simulink subsystem "propagation"  (R2023b)
settings: Solver=VariableStepAuto  StartTime=0.0  StopTime=10.0  RelTol=1e-3
undefined symbols (not defined in the file or in its folder): P0, Propagation, R_sensor2body, x0
undefined symbols (not defined in the file): states_k
libraries: nav_lib x7
settings Model: Creator=brent  LastModifiedBy=brent

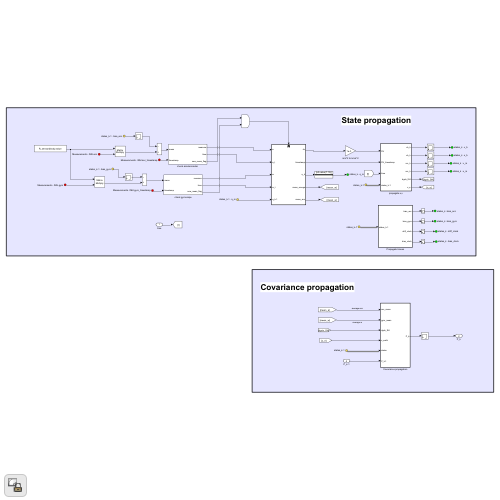
[thumbnail: Simulink's stored preview of the top-level diagram]
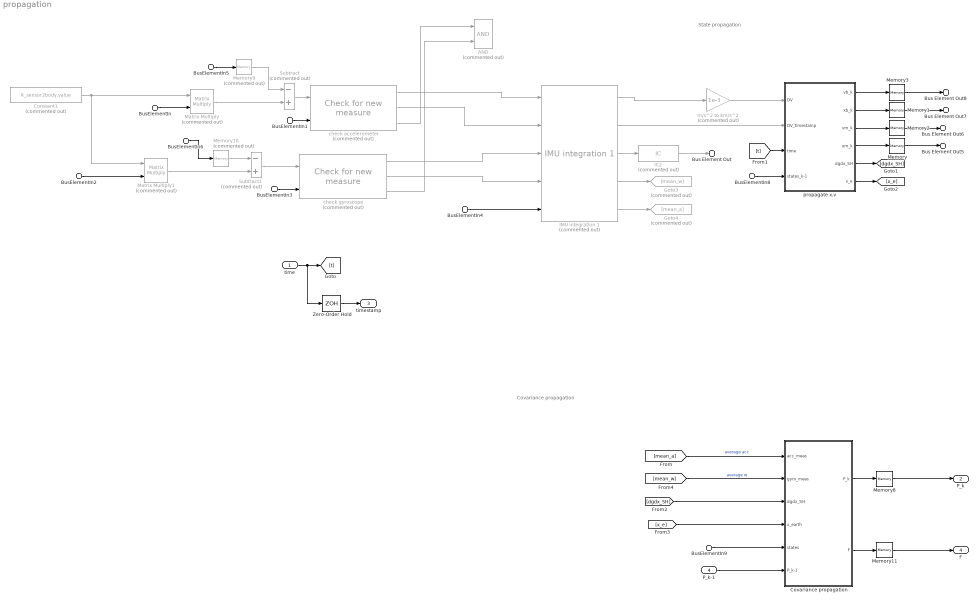
== system propagation ==
  note: State propagation
  note: Covariance propagation
  time : Inport
  BusElementIn1 : Inport  Port=2  PortName=Measurements  Element=IMU.acc_timestamp
  BusElementIn3 : Inport  Port=2  PortName=Measurements  Element=IMU.gyro_timestamp
  BusElementIn : Inport  Port=2  PortName=Measurements  Element=IMU.acc
  BusElementIn2 : Inport  Port=2  PortName=Measurements  Element=IMU.gyro
  BusElementIn8 : Inport  Port=3  PortName=states_k-1
  BusElementIn9 : Inport  Port=3  PortName=states_k-1
  BusElementIn4 : Inport  Port=3  PortName=states_k-1  Element=q_m
  BusElementIn5 : Inport  Port=3  PortName=states_k-1  Element=bias_acc
  BusElementIn6 : Inport  Port=3  PortName=states_k-1  Element=bias_gyro
  P_k-1 : Inport  Port=4
  AND : Logic  Commented=on  IconShape=distinctive  AllPortsSameDT=off  OutDataTypeStr=boolean
  Constant1 : Constant  Commented=on  Value=R_sensor2body.value
  Covariance propagation : Subsystem  TreatAsAtomicUnit=on  SystemSampleTime=1/Propagation.lf.value
  Goto3 : Goto  Commented=on  GotoTag=mean_w
  Goto4 : Goto  Commented=on  GotoTag=mean_a
  IC2 : InitialCondition  Commented=on  Value=x0.value(7:10)
  IMU integration 1 : nav_lib/IMU integration 1  Commented=on  q0=x0.value(7:10)  HF=Propagation.hf.value  LF=Propagation.lf.value
      settings: SourceProductName=Navigation library
  Matrix Multiply : Product  Commented=on  Multiplication=Matrix(*)
  Matrix Multiply1 : Product  Commented=on  Multiplication=Matrix(*)
  Memory : Memory  InitialCondition=x0.value(1:3)  InheritSampleTime=on
  Memory1 : Memory  InitialCondition=x0.value(11:13)  InheritSampleTime=on
  Memory10 : Memory  Commented=on  InitialCondition=x0.value(20:22)
  Memory11 : Memory  InitialCondition=eye(12)  InheritSampleTime=on
  Memory2 : Memory  InitialCondition=x0.value(4:6)  InheritSampleTime=on
  Memory3 : Memory  InitialCondition=x0.value(14:16)  InheritSampleTime=on
  Memory8 : Memory  InitialCondition=P0.value([1:6 10:15],[1:6 10:15])  InheritSampleTime=on
  Memory9 : Memory  Commented=on  InitialCondition=x0.value(17:19)
  Subtract : Sum  Commented=on  Inputs=-+
  Subtract1 : Sum  Commented=on  Inputs=-+
  Zero-Order Hold : ZeroOrderHold  SampleTime=1/Propagation.lf.value
  check accelerometer : nav_lib/Check for new measure  Commented=on  Ts=1/Propagation.hf.value
      settings: SourceProductName=Navigation library
  check gyroscope : nav_lib/Check for new measure  Commented=on  Ts=1/Propagation.hf.value
      settings: SourceProductName=Navigation library
  m/s^2 to km/s^2 : Gain  Commented=on  Gain=1e-3
  propagate x,v : Subsystem  TreatAsAtomicUnit=on  SystemSampleTime=1/Propagation.lf.value
  Bus Element Out5 : Outport  PortName=states_k  Element=x_m
  Bus Element Out6 : Outport  PortName=states_k  Element=v_m
  Bus Element Out : Outport  PortName=states_k  Element=q_m
  Bus Element Out7 : Outport  PortName=states_k  Element=x_b
  Bus Element Out8 : Outport  PortName=states_k  Element=v_b
  P_k : Outport  Port=2
  timestamp : Outport  Port=3
  F : Outport  Port=4
  wires:
  BusElementIn1/1 -> check accelerometer/2
  BusElementIn3/1 -> check gyroscope/2
  check accelerometer/3 -> AND/1
  check gyroscope/3 -> AND/2
  time/1 -> [t], Zero-Order Hold/1
  BusElementIn/1 -> Matrix Multiply/2
  Constant1/1 -> Matrix Multiply1/1, Matrix Multiply/1
  BusElementIn2/1 -> Matrix Multiply1/2
  Matrix Multiply/1 -> Subtract/2
  Subtract/1 -> check accelerometer/1
  BusElementIn5/1 -> Memory9/1
  m/s^2 to km/s^2/1 -> propagate x,v/1(DV)
  Subtract1/1 -> check gyroscope/1
  BusElementIn6/1 -> Memory10/1
  Matrix Multiply1/1 -> Subtract1/2
  [t] -> propagate x,v/3(time)
  BusElementIn8/1 -> propagate x,v/4(states_k-1)
  propagate x,v/4(xm_k) -> Memory/1
  propagate x,v/3(vm_k) -> Memory2/1
  propagate x,v/2(xb_k) -> Memory1/1
  propagate x,v/1(vb_k) -> Memory3/1
  Memory1/1 -> Bus Element Out7/1
  Memory/1 -> Bus Element Out5/1
  Memory2/1 -> Bus Element Out6/1
  Memory3/1 -> Bus Element Out8/1
  BusElementIn4/1 -> IMU integration 1/5
  IC2/1 -> Bus Element Out/1
  propagate x,v/5(dgdx_SH) -> [dgdx_SH]
  propagate x,v/6(x_e) -> [x_e]
  [dgdx_SH] -> Covariance propagation/3(dgdx_SH)
  [x_e] -> Covariance propagation/4(x_earth)
  BusElementIn9/1 -> Covariance propagation/5(states)
  P_k-1/1 -> Covariance propagation/6(P_k-1)
  IMU integration 1/4 -> Goto3/1
  [mean_w] -> Covariance propagation/2(gyro_meas)  "average w"
  [mean_a] -> Covariance propagation/1(acc_meas)  "average acc"
  check accelerometer/1 -> IMU integration 1/1
  check accelerometer/2 -> IMU integration 1/2
  check gyroscope/1 -> IMU integration 1/3
  check gyroscope/2 -> IMU integration 1/4
  IMU integration 1/1 -> m/s^2 to km/s^2/1
  IMU integration 1/3 -> IC2/1
  IMU integration 1/2 -> propagate x,v/2(DV_timestamp)
  IMU integration 1/5 -> Goto4/1
  Covariance propagation/1(P_k) -> Memory8/1
  Memory8/1 -> P_k/1
  Memory9/1 -> Subtract/1
  Memory10/1 -> Subtract1/1
  Zero-Order Hold/1 -> timestamp/1
  Covariance propagation/2(F) -> Memory11/1
  Memory11/1 -> F/1

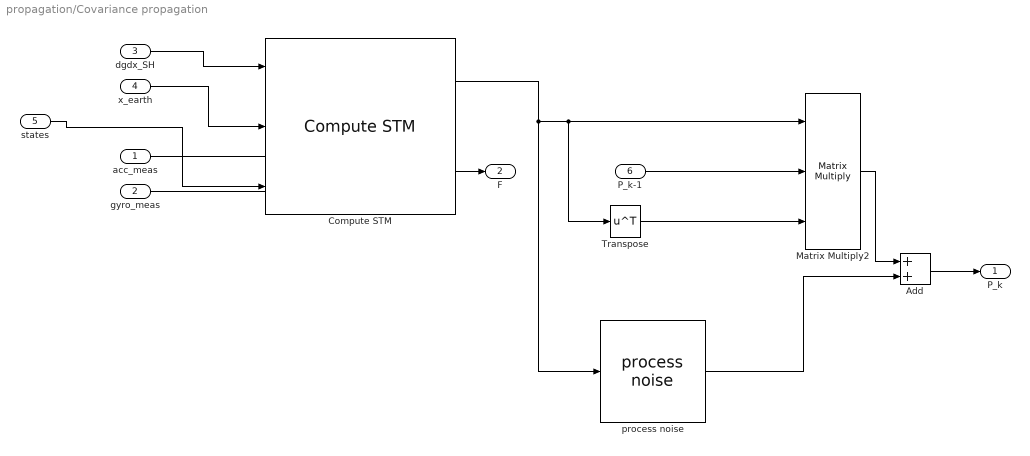
== system propagation/Covariance propagation ==
  acc_meas : Inport
  gyro_meas : Inport  Port=2
  dgdx_SH : Inport  Port=3
  x_earth : Inport  Port=4
  states : Inport  Port=5
  P_k-1 : Inport  Port=6
  Add : Sum
  Compute STM : nav_lib/Compute STM  dt=1/Propagation.lf.value  mu_e=Propagation.Earth.mu.value  mu_m=Propagation.Moon.mu.value  x0=x0.value
      settings: SourceProductName=Navigation library
  Matrix Multiply2 : Product  Inputs=3  Multiplication=Matrix(*)
  Transpose : Math  Operator=transpose
  process noise : nav_lib/process noise  Q=Q.value  R_sb=R_sensor2body.value  dt=1/Propagation.lf.value
      settings: SourceProductName=Navigation library
  P_k : Outport
  F : Outport  Port=2
  wires:
  process noise/1 -> Add/2
  Compute STM/2 -> F/1
  Add/1 -> P_k/1
  Matrix Multiply2/1 -> Add/1
  Compute STM/1 -> Transpose/1, Matrix Multiply2/1, process noise/1
  states/1 -> Compute STM/3
  x_earth/1 -> Compute STM/2
  dgdx_SH/1 -> Compute STM/1
  Transpose/1 -> Matrix Multiply2/3
  P_k-1/1 -> Matrix Multiply2/2
  gyro_meas/1 -> ?
  acc_meas/1 -> ?

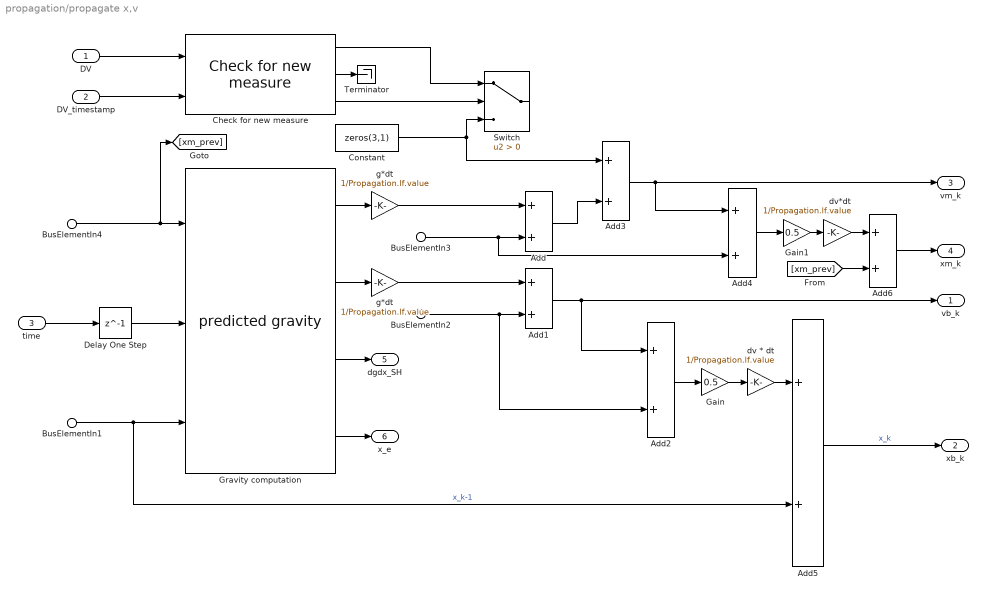
== system propagation/propagate x,v ==
  DV : Inport
  DV_timestamp : Inport  Port=2
  time : Inport  Port=3
  BusElementIn4 : Inport  Port=4  PortName=states_k-1  Element=x_m
  BusElementIn3 : Inport  Port=4  PortName=states_k-1  Element=v_m
  BusElementIn1 : Inport  Port=4  PortName=states_k-1  Element=x_b
  BusElementIn2 : Inport  Port=4  PortName=states_k-1  Element=v_b
  Add{,1..6} (7 alike) : Sum
  Check for new measure : nav_lib/Check for new measure  Ts=0
      settings: SourceProductName=Navigation library
  Constant : Constant  Value=zeros(3,1)  VectorParams1D=off
  Delay One Step : Delay  DelayLength=1
  Gain : Gain  Gain=0.5
  Gain1 : Gain  Gain=0.5
  Gravity computation : nav_lib/predicted gravity  date=StartDate  Earth=Propagation.Earth  Moon=Propagation.Moon
      settings: SourceProductName=Navigation library
  Switch : Switch  Criteria=u2 > Threshold  SaturateOnIntegerOverflow=off  InputSameDT=off
  Terminator : Terminator
  dv * dt : Gain  Gain=1/Propagation.lf.value
  dv*dt : Gain  Gain=1/Propagation.lf.value
  g*dt : Gain  Gain=1/Propagation.lf.value
  "g*dt " : Gain  Gain=1/Propagation.lf.value
  vb_k : Outport
  xb_k : Outport  Port=2
  vm_k : Outport  Port=3
  xm_k : Outport  Port=4
  dgdx_SH : Outport  Port=5
  x_e : Outport  Port=6
  wires:
  Delay One Step/1 -> Gravity computation/2
  dv*dt/1 -> Add6/1
  Gain1/1 -> dv*dt/1
  dv * dt/1 -> Add5/1
  Gravity computation/4 -> x_e/1
  Gravity computation/3 -> dgdx_SH/1
  Add6/1 -> xm_k/1
  [xm_prev] -> Add6/2
  Add5/1 -> xb_k/1  "x_k"
  Gain/1 -> dv * dt/1
  BusElementIn1/1 -> Add5/2, Gravity computation/3  "x_k-1"
  BusElementIn4/1 -> Gravity computation/1, [xm_prev]
  time/1 -> Delay One Step/1
  Add4/1 -> Gain1/1
  BusElementIn3/1 -> Add/2, Add4/2
  Add3/1 -> vm_k/1, Add4/1
  "g*dt "/1 -> Add/1
  Constant/1 -> Switch/3, Add3/1
  Check for new measure/1 -> Switch/1
  Add/1 -> Add3/2
  Add2/1 -> Gain/1
  BusElementIn2/1 -> Add1/2, Add2/2
  Add1/1 -> vb_k/1, Add2/1
  Check for new measure/3 -> Switch/2
  g*dt/1 -> Add1/1
  Gravity computation/2 -> g*dt/1
  Gravity computation/1 -> "g*dt "/1
  Check for new measure/2 -> Terminator/1
  DV_timestamp/1 -> Check for new measure/2
  DV/1 -> Check for new measure/1
